simulink model "MCC_retour_etat_estime"  (R2024a)
settings: Solver=ode45  StartTime=0.0  StopTime=Tfinal  RelTol=1e-3
undefined symbols (not defined in the file): A, B_sim, C, C_obs, D_obs, D_sim, K, Nr, Tmec, x0
settings Model: Creator=DELL  LastModifiedBy=DELL

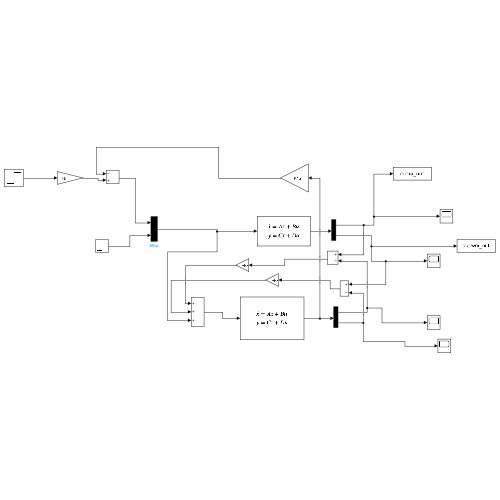
[thumbnail: Simulink's stored preview of the top-level diagram]
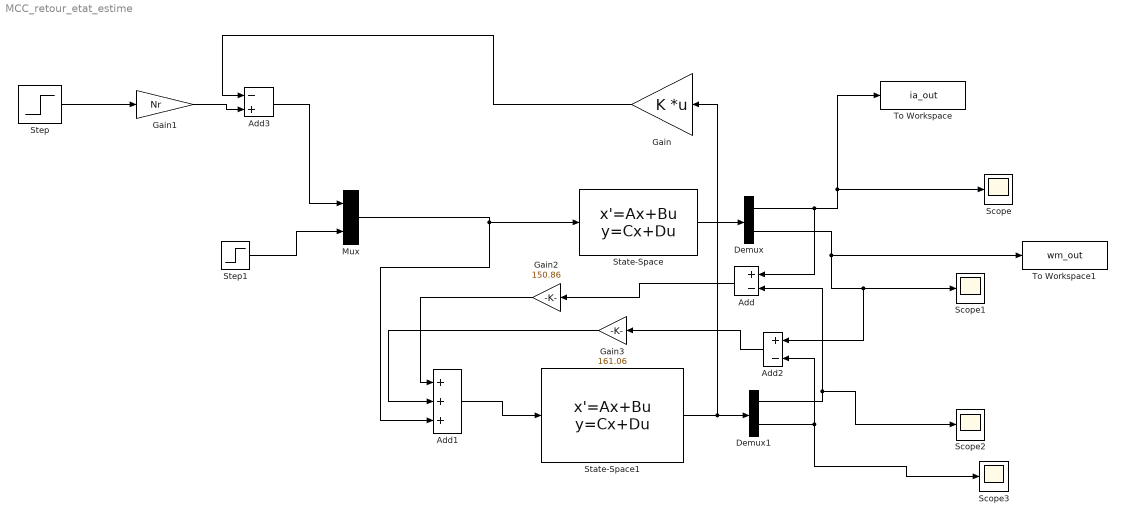
== system MCC_retour_etat_estime ==
  Add : Sum  Inputs=+-
  Add1 : Sum  Inputs=+++
  Add2 : Sum  Inputs=+-
  Add3 : Sum  Inputs=-+
  Demux : Demux  Outputs=2
  Demux1 : Demux  Outputs=2
  Gain : Gain  Gain=K  Multiplication=Matrix(K*u)
  Gain1 : Gain  Gain=Nr
  Gain2 : Gain  Gain=150.86
  Gain3 : Gain  Gain=161.06
  Mux : Mux  Inputs=2
  Scope{,1..3} (4 alike) : Scope
  State-Space : StateSpace  A=A  B=B_sim  C=C  D=D_sim  InitialCondition=x0
  State-Space1 : StateSpace  A=A  B=B_sim  C=C_obs  D=D_obs  InitialCondition=x0
  Step : Step  Time=0.1  After=100  SampleTime=0
  Step1 : Step  Time=0.5  After=Tmec  SampleTime=0
  To Workspace : ToWorkspace  VariableName=ia_out  SaveFormat=Timeseries  SampleTime=-1
  To Workspace1 : ToWorkspace  VariableName=wm_out  SaveFormat=Timeseries  SampleTime=-1
  wires:
  Mux/1 -> State-Space/1, Add1/3
  Step1/1 -> Mux/2
  Demux/1 -> Add/1, Scope/1, To Workspace/1
  Demux/2 -> Add2/1, Scope1/1, To Workspace1/1
  Add3/1 -> Mux/1
  Gain/1 -> Add3/1
  State-Space/1 -> Demux/1
  Step/1 -> Gain1/1
  Gain1/1 -> Add3/2
  Add/1 -> Gain2/1
  Add1/1 -> State-Space1/1
  State-Space1/1 -> Gain/1, Demux1/1
  Demux1/1 -> Add/2, Scope2/1
  Demux1/2 -> Scope3/1, Add2/2
  Add2/1 -> Gain3/1
  Gain3/1 -> Add1/2
  Gain2/1 -> Add1/1
